simulink model "sampleModel2067"  (R2023a)
settings: Solver=VariableStepAuto  StartTime=0.0  StopTime=10.0  RelTol=1e-3
libraries: hdlsllib x5, simulink x4
settings Model: Creator=user1  LastModifiedBy=user1

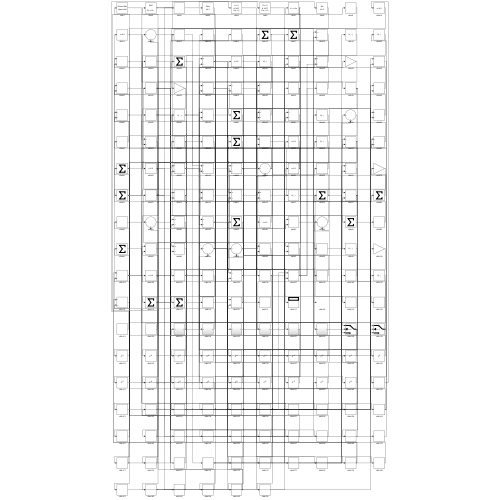
[thumbnail: Simulink's stored preview of the top-level diagram]
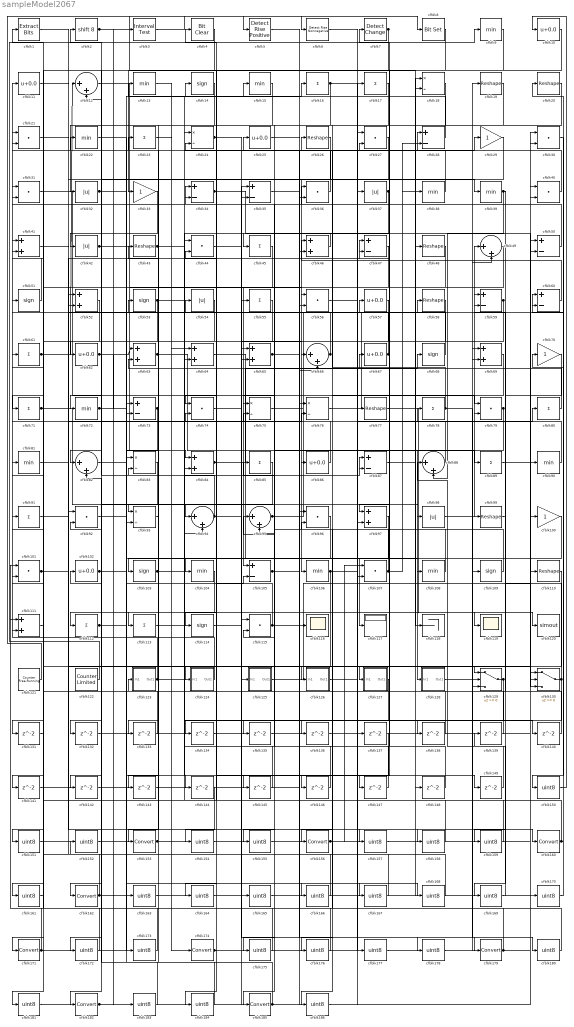
== system sampleModel2067 ==
  cfblk1 : simulink/Logic and Bit Operations/Extract Bits  bitsToExtract=Upper half  numBits=8  bitIdxRange=[0 7]  outScalingMode=Preserve fixed-point scaling
      settings: LibrarySourceBlock=|
      | hdlsllib/Logic and Bit
      | Operations/Extract Bits
  cfblk{10..11,25,57,62,67,86,102} (8 alike) : Bias  Bias=0.0  SaturateOnIntegerOverflow=off
  cfblk{29,33,70,100} (4 alike) : Gain
  cfblk{21,27,30..31,36,40,44,56,74,79,92,96,101,107,115} (15 alike) : DotProduct  OutDataTypeStr=Inherit: Inherit via internal rule
  cfblk{14,51,53,68,103,109,114} (7 alike) : Signum
  cfblk{9,13,15,22,38..39,72,81,90,104,106,108} (12 alike) : MinMax
  cfblk{28,34..35,47,50,59..60,73,87,105} (10 alike) : Sum  Inputs=+-
  cfblk{19..20,26,43,48,58,77,99,110} (9 alike) : Reshape
  cfblk{41,46,52,63..65,69,84,97,111} (10 alike) : Sum
  cfblk{16..17,23,45,55,61,71,78,80,85,89,91,112..113} (14 alike) : Sum  Inputs=+
  cfblk116 : Scope
  cfblk117 : Display
  cfblk118 : Terminator
  cfblk119 : Scope
  cfblk{12,49,66,82,88,94..95} (7 alike) : Sum  Inputs=|++
  cfblk120 : ToWorkspace  VariableName=simout  SaveFormat=Timeseries  SampleTime=-1
  cfblk121 : hdlsllib/Sources/Counter Free-Running  NumBits=16  tsamp=-1
  cfblk122 : hdlsllib/Sources/Counter Limited  uplimit=7  tsamp=-1
  cfblk123 : Subsystem
      settings: LibrarySourceBlock=|
      | hdlsllib/Ports &
      | Subsystems/Subsystem
  cfblk124 : Subsystem
      settings: LibrarySourceBlock=|
      | hdlsllib/Ports &
      | Subsystems/Subsystem
  cfblk125 : Subsystem
      settings: LibrarySourceBlock=|
      | hdlsllib/Ports &
      | Subsystems/Subsystem
  cfblk126 : Subsystem
      settings: LibrarySourceBlock=|
      | hdlsllib/Ports &
      | Subsystems/Subsystem
  cfblk127 : Subsystem
      settings: LibrarySourceBlock=|
      | hdlsllib/Ports &
      | Subsystems/Subsystem
  cfblk128 : Subsystem
      settings: LibrarySourceBlock=|
      | hdlsllib/Ports &
      | Subsystems/Subsystem
  cfblk129 : Switch  SaturateOnIntegerOverflow=off  InputSameDT=off
  cfblk130 : Switch  SaturateOnIntegerOverflow=off  InputSameDT=off
  cfblk{131..149} (19 alike) : Delay  SampleTime=1
  cfblk{150..152,154..155,157..159,161,163..170,172..173,175..178,180..181,183..184,186} (28 alike) : DataTypeConversion  OutDataTypeStr=uint8  SaturateOnIntegerOverflow=off  RndMeth=Floor
  cfblk{153,156,160,162,171,174,179,182,185} (9 alike) : DataTypeConversion  SaturateOnIntegerOverflow=off  RndMeth=Floor
  cfblk{18,24,75..76,83,93} (6 alike) : Product  Inputs=*/  RndMeth=Zero  SaturateOnIntegerOverflow=on
  cfblk2 : ArithShift  BitShiftNumber=8
  cfblk3 : hdlsllib/Logic and Bit Operations/Interval Test  IntervalClosedRight=on  uplimit=0.5  IntervalClosedLeft=on  lowlimit=-0.5  OutDataTypeStr=boolean
  cfblk{32,37,42,54,98} (5 alike) : Abs  SaturateOnIntegerOverflow=off
  cfblk4 : simulink/Logic and Bit Operations/Bit Clear  iBit=0
      settings: LibrarySourceBlock=|
      | hdlsllib/Logic and Bit
      | Operations/Bit Clear
  cfblk5 : hdlsllib/Logic and Bit Operations/Detect Rise Positive  vinit=0  OutDataTypeStr=boolean
  cfblk6 : hdlsllib/Logic and Bit Operations/Detect Rise Nonnegative  vinit=0  OutDataTypeStr=boolean
  cfblk7 : simulink/Logic and Bit Operations/Detect Change  vinit=0  OutDataTypeStr=boolean
      settings: LibrarySourceBlock=|
      | hdlsllib/Logic and Bit
      | Operations/Detect
      | Change
  cfblk8 : simulink/Logic and Bit Operations/Bit Set  iBit=0
      settings: LibrarySourceBlock=|
      | hdlsllib/Logic and Bit
      | Operations/Bit Set
  wires:
  cfblk79/1 -> cfblk11/1, cfblk155/1
  cfblk47/1 -> cfblk105/1
  cfblk13/1 -> cfblk64/1
  cfblk76/1 -> cfblk20/1
  cfblk42/1 -> cfblk84/1, cfblk107/2
  cfblk84/1 -> cfblk67/1, cfblk127/1(In1)
  cfblk17/1 -> cfblk185/1
  cfblk129/1 -> cfblk134/1, cfblk135/1
  cfblk98/1 -> cfblk49/1
  cfblk123/1(Out1) -> cfblk21/1, cfblk16/1
  cfblk64/1 -> cfblk117/1
  cfblk122/1 -> cfblk9/1
  cfblk31/1 -> cfblk79/1
  cfblk27/1 -> cfblk94/1
  cfblk63/1 -> cfblk128/1(In1), cfblk120/1
  cfblk124/1(Out1) -> cfblk113/1
  cfblk9/1 -> cfblk97/1
  cfblk61/1 -> cfblk12/1, cfblk181/1
  cfblk15/1 -> cfblk124/1(In1)
  cfblk26/1 -> cfblk106/1
  cfblk112/1 -> cfblk15/1, cfblk105/2
  cfblk12/1 -> cfblk56/1
  cfblk75/1 -> cfblk58/1
  cfblk111/1 -> cfblk171/1
  cfblk46/1 -> cfblk45/1
  cfblk43/1 -> cfblk29/1, cfblk138/1
  cfblk95/1 -> cfblk68/1, cfblk66/2
  cfblk11/1 -> cfblk52/1
  cfblk62/1 -> cfblk63/1, cfblk163/1
  cfblk80/1 -> cfblk63/2
  cfblk35/1 -> cfblk179/1
  cfblk7/1 -> cfblk33/1, cfblk46/2
  cfblk114/1 -> cfblk57/1
  cfblk99/1 -> cfblk123/1(In1)
  cfblk125/1(Out1) -> cfblk90/1
  cfblk102/1 -> cfblk129/2, cfblk167/1
  cfblk73/1 -> cfblk53/1, cfblk93/2
  cfblk65/1 -> cfblk28/1, cfblk60/1, cfblk175/1
  cfblk53/1 -> cfblk103/1, cfblk25/1, cfblk142/1
  cfblk107/1 -> cfblk31/1, cfblk38/1, cfblk28/2
  cfblk68/1 -> cfblk2/1
  cfblk77/1 -> cfblk119/1
  cfblk86/1 -> cfblk14/1
  cfblk28/1 -> cfblk13/1
  cfblk83/1 -> cfblk182/1
  cfblk115/1 -> cfblk54/1, cfblk87/2
  cfblk55/1 -> cfblk162/1
  cfblk14/1 -> cfblk32/1
  cfblk89/1 -> cfblk50/1
  cfblk18/1 -> cfblk153/1
  cfblk72/1 -> cfblk22/1, cfblk3/1, cfblk144/1, cfblk183/1
  cfblk128/1(Out1) -> cfblk19/1
  cfblk91/1 -> cfblk160/1
  cfblk37/1 -> cfblk75/1, cfblk64/2
  cfblk103/1 -> cfblk87/1, cfblk140/1
  cfblk36/1 -> cfblk21/2
  cfblk66/1 -> cfblk34/1, cfblk41/2
  cfblk40/1 -> cfblk27/2
  cfblk109/1 -> cfblk85/1
  cfblk82/1 -> cfblk76/2
  cfblk108/1 -> cfblk51/1
  cfblk60/1 -> cfblk46/1
  cfblk21/1 -> cfblk52/2
  cfblk90/1 -> cfblk7/1
  cfblk67/1 -> cfblk36/1, cfblk43/1
  cfblk71/1 -> cfblk125/1(In1), cfblk47/1
  cfblk38/1 -> cfblk26/1
  cfblk126/1(Out1) -> cfblk77/1
  cfblk121/1 -> cfblk8/1
  cfblk87/1 -> cfblk89/1
  cfblk34/1 -> cfblk130/1, cfblk178/1
  cfblk20/1 -> cfblk86/1
  cfblk88/1 -> cfblk78/1
  cfblk130/1 -> cfblk59/2, cfblk186/1
  cfblk58/1 -> cfblk62/1
  cfblk50/1 -> cfblk4/1
  cfblk16/1 -> cfblk95/2, cfblk130/3
  cfblk105/1 -> cfblk36/2, cfblk75/2
  cfblk23/1 -> cfblk174/1
  cfblk56/1 -> cfblk97/2
  cfblk3/1 -> cfblk5/1
  cfblk39/1 -> cfblk88/2, cfblk159/1
  cfblk32/1 -> cfblk129/3, cfblk84/2, cfblk168/1
  cfblk2/1 -> cfblk6/1, cfblk118/1
  cfblk1/1 -> cfblk39/1
  cfblk24/1 -> cfblk65/2, cfblk66/1
  cfblk94/1 -> cfblk12/2, cfblk108/1, cfblk98/1, cfblk146/1
  cfblk106/1 -> cfblk126/1(In1), cfblk80/1
  cfblk5/1 -> cfblk50/2
  cfblk100/1 -> cfblk156/1
  cfblk85/1 -> cfblk93/1
  cfblk8/1 -> cfblk42/1
  cfblk25/1 -> cfblk116/1
  cfblk101/1 -> cfblk59/1, cfblk74/2
  cfblk49/1 -> cfblk82/1
  cfblk59/1 -> cfblk74/1, cfblk136/1
  cfblk29/1 -> cfblk72/1
  cfblk78/1 -> cfblk24/2, cfblk180/1
  cfblk57/1 -> cfblk112/1
  cfblk96/1 -> cfblk104/1
  cfblk48/1 -> cfblk71/1
  cfblk41/1 -> cfblk129/1
  cfblk51/1 -> cfblk41/1
  cfblk10/1 -> cfblk114/1
  cfblk52/1 -> cfblk131/1
  cfblk131/1 -> cfblk1/1
  cfblk104/1 -> cfblk132/1
  cfblk132/1 -> cfblk65/1
  cfblk97/1 -> cfblk133/1
  cfblk133/1 -> cfblk31/2
  cfblk134/1 -> cfblk27/1
  cfblk135/1 -> cfblk130/2
  cfblk136/1 -> cfblk49/2
  cfblk138/1 -> cfblk115/2
  cfblk139/1 -> cfblk82/2
  cfblk140/1 -> cfblk79/2
  cfblk4/1 -> cfblk141/1
  cfblk141/1 -> cfblk76/1
  cfblk142/1 -> cfblk73/1
  cfblk93/1 -> cfblk143/1
  cfblk143/1 -> cfblk94/2
  cfblk127/1(Out1) -> cfblk145/1
  cfblk145/1 -> cfblk24/1
  cfblk146/1 -> cfblk34/2
  cfblk19/1 -> cfblk147/1
  cfblk147/1 -> cfblk95/1
  cfblk148/1 -> cfblk47/2
  cfblk113/1 -> cfblk149/1
  cfblk149/1 -> cfblk88/1
  cfblk30/1 -> cfblk150/1
  cfblk150/1 -> cfblk10/1
  cfblk110/1 -> cfblk151/1
  cfblk151/1 -> cfblk30/1
  cfblk152/1 -> cfblk30/2
  cfblk153/1 -> cfblk109/1, cfblk40/2
  cfblk144/1 -> cfblk154/1
  cfblk154/1 -> cfblk18/1
  cfblk155/1 -> cfblk18/2
  cfblk156/1 -> cfblk48/1, cfblk107/1
  cfblk44/1 -> cfblk157/1
  cfblk157/1 -> cfblk100/1
  cfblk81/1 -> cfblk158/1
  cfblk158/1 -> cfblk44/1
  cfblk159/1 -> cfblk81/1
  cfblk160/1 -> cfblk60/2, cfblk44/2
  cfblk54/1 -> cfblk161/1
  cfblk161/1 -> cfblk91/1
  cfblk162/1 -> cfblk148/1, cfblk61/1
  cfblk163/1 -> cfblk55/1
  cfblk137/1 -> cfblk164/1
  cfblk164/1 -> cfblk40/1
  cfblk74/1 -> cfblk165/1
  cfblk165/1 -> cfblk137/1
  cfblk92/1 -> cfblk166/1
  cfblk166/1 -> cfblk101/2
  cfblk167/1 -> cfblk92/1
  cfblk168/1 -> cfblk92/2
  cfblk70/1 -> cfblk169/1
  cfblk169/1 -> cfblk139/1
  cfblk170/1 -> cfblk70/1
  cfblk171/1 -> cfblk73/2, cfblk101/1
  cfblk33/1 -> cfblk172/1
  cfblk172/1 -> cfblk111/1
  cfblk22/1 -> cfblk173/1
  cfblk173/1 -> cfblk111/2
  cfblk174/1 -> cfblk37/1, cfblk110/1, cfblk99/1
  cfblk175/1 -> cfblk23/1
  cfblk69/1 -> cfblk176/1
  cfblk176/1 -> cfblk96/1
  cfblk6/1 -> cfblk177/1
  cfblk177/1 -> cfblk69/1
  cfblk178/1 -> cfblk69/2
  cfblk179/1 -> cfblk96/2, cfblk102/1
  cfblk180/1 -> cfblk35/1
  cfblk181/1 -> cfblk35/2
  cfblk182/1 -> cfblk170/1, cfblk56/2
  cfblk183/1 -> cfblk83/1
  cfblk45/1 -> cfblk184/1
  cfblk184/1 -> cfblk83/2
  cfblk185/1 -> cfblk152/1, cfblk115/1
  cfblk186/1 -> cfblk17/1

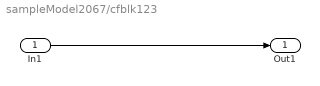
== system sampleModel2067/cfblk123 ==
  In1 : Inport
  Out1 : Outport
  wires:
  In1/1 -> Out1/1

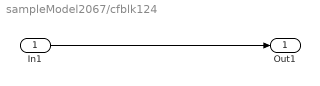
== system sampleModel2067/cfblk124 ==
  In1 : Inport
  Out1 : Outport
  wires:
  In1/1 -> Out1/1

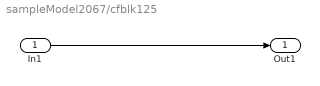
== system sampleModel2067/cfblk125 ==
  In1 : Inport
  Out1 : Outport
  wires:
  In1/1 -> Out1/1

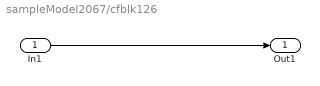
== system sampleModel2067/cfblk126 ==
  In1 : Inport
  Out1 : Outport
  wires:
  In1/1 -> Out1/1

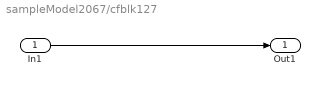
== system sampleModel2067/cfblk127 ==
  In1 : Inport
  Out1 : Outport
  wires:
  In1/1 -> Out1/1

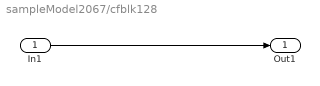
== system sampleModel2067/cfblk128 ==
  In1 : Inport
  Out1 : Outport
  wires:
  In1/1 -> Out1/1
